simulink model "TZ_H2zsimulink"  (R2021b)
settings: Solver=FixedStepDiscrete  StartTime=0.0  StopTime=10.0  FixedStep=Ts  RelTol=1e-3
libraries: cstblocks x4
settings Model: Creator=3711538  LastModifiedBy=sarmeegan
settings SolverCC: AlgebraicLoopSolver=TrustRegion
settings DebuggingCC: SFMachineParentedDataDiag=warning
settings SFSimCC: CustomCodeUndefinedFunction=UseInterfaceOnly

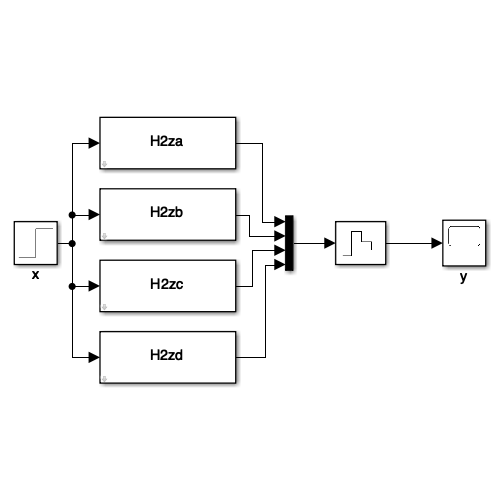
[thumbnail: Simulink's stored preview of the top-level diagram]
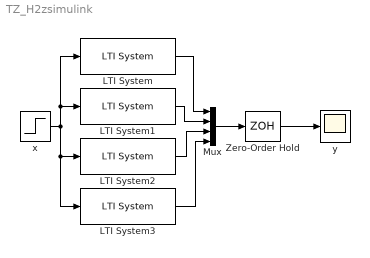
== system TZ_H2zsimulink ==
  LTI System : cstblocks/LTI System  sys=H2za  IC=[]
  LTI System1 : cstblocks/LTI System  sys=H2zb  IC=[]
  LTI System2 : cstblocks/LTI System  sys=H2zc  IC=[]
  LTI System3 : cstblocks/LTI System  sys=H2zd  IC=[]
  Mux : Mux
  Zero-Order Hold : ZeroOrderHold  SampleTime=-1
  x : Step  SampleTime=0
  y : Scope
  wires:
  Zero-Order Hold/1 -> y/1
  x/1 -> LTI System3/1, LTI System2/1, LTI System1/1, LTI System/1
  LTI System/1 -> Mux/1
  LTI System1/1 -> Mux/2
  LTI System2/1 -> Mux/3
  LTI System3/1 -> Mux/4
  Mux/1 -> Zero-Order Hold/1
